simulink model "Model_FOPID_autotuning"  (Simulink 9.2)
settings: Solver=VariableStepAuto  StartTime=0.0  StopTime=100  FixedStep=T_s  MaxStep=1e-3  RelTol=1e-3  EnableMultiTasking=on
values from neighbouring files (symbols this model uses):
  d = step_value    (= 1)    [GUI_ZNFOPID.m]
  disturb_step_time = sim_time*2    (= 200)    [GUI_ZNFOPID.m]
  disturb_step_value = 0.3    [GUI_ZNFOPID.m]
  h = step_value    (= 1)    [GUI_ZNFOPID.m]
  Kp = alpha*Kc    [Function_ZNPID_mu.m]    (also in GUI_ZNFOPID.m = handles.Kp)
  L = 0    [GUI_ZNFOPID.m]
  step_value = 1    [GUI_ZNFOPID.m]
  SW = 0    [GUI_ZNFOPID.m]
  Td = gamma*Tc^mu    [Function_ZNPID_mu.m]    (also in GUI_ZNFOPID.m = handles.Td)
  Ti = beta*Tc    [Function_ZNPID_mu.m]    (also in GUI_ZNFOPID.m = handles.Ti)
libraries: cstblocks x2, powerlib x1
settings Model: Creator=Li Chuang  LastModifiedBy=18764
settings OptimizationCC: InitFltsAndDblsToZero=on
settings DebuggingCC: SaveWithParameterizedLinksMsg=none  SignalResolutionControl=TryResolveAllWithWarning  SolverPrmCheckMsg=warning  MultiTaskDSMMsg=warning  MultiTaskCondExecSysMsg=none  FcnCallInpInsideContextMsg=error  AllowSymbolicDim=off  StateNameClashWarn=none
settings GRTTargetCC: TargetFcnLib=ansi_tfl_tmw.mat  GeneratePreprocessorConditionals=Use local settings

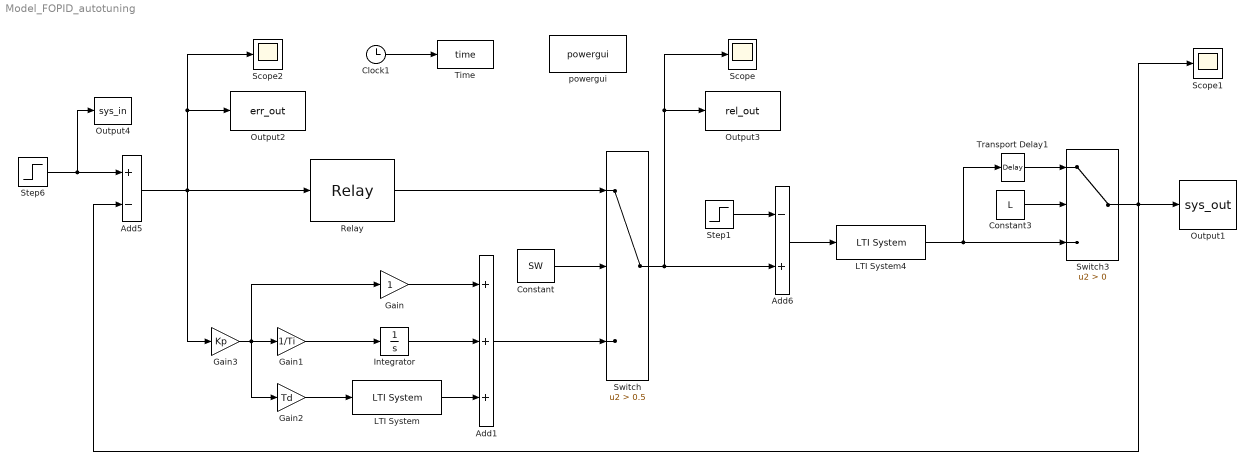
== system Model_FOPID_autotuning ==
  Add1 : Sum  Inputs=+++  SaturateOnIntegerOverflow=on  OutDataTypeStr=Inherit: Same as first input
  Add5 : Sum  Inputs=+-  SaturateOnIntegerOverflow=on  OutDataTypeStr=Inherit: Same as first input
  Add6 : Sum  Inputs=-+  SaturateOnIntegerOverflow=on  OutDataTypeStr=Inherit: Same as first input
  Clock1 : Clock
      settings: Decimation=100
  Constant : Constant  Value=SW
  Constant3 : Constant  Value=L
  Gain : Gain
  Gain1 : Gain  Gain=1/Ti
  Gain2 : Gain  Gain=Td
  Gain3 : Gain  Gain=Kp
  Integrator : Integrator
  LTI System : cstblocks/LTI System  sys=dfo  IC=[]
  LTI System4 : cstblocks/LTI System  sys=Gp  IC=[]
  Output1 : ToWorkspace  VariableName=sys_out  SampleTime=-1
  Output2 : ToWorkspace  VariableName=err_out  SampleTime=-1
  Output3 : ToWorkspace  VariableName=rel_out  SampleTime=-1
  Output4 : ToWorkspace  VariableName=sys_in  SampleTime=-1
  Relay : Relay  OnSwitchValue=d  OffSwitchValue=-d  OnOutputValue=h  OffOutputValue=-h
  Scope : Scope
  Scope1 : Scope
  Scope2 : Scope
  Step1 : Step  Time=disturb_step_time  After=disturb_step_value
  Step6 : Step  Time=0  After=step_value
  Switch : Switch  Criteria=u2 > Threshold  Threshold=0.5
  Switch3 : Switch  Criteria=u2 > Threshold
  Time : ToWorkspace  VariableName=time  SampleTime=-1
  Transport Delay1 : TransportDelay  DelayTime=L
  powergui : powerlib/powergui  Priority=1  SimulationMode=Continuous  SampleTime=50e-6  frequency=60  Iterations=50  frequencyindice=60  Pbase=100e6  ErrMax=1e-4  UnitsV=kV  UnitsW=MW  buscounter=0  FunctionMessages=off  echomessages=off  EnableUseOfTLC=off  CurrentSourceSwitches=off  DisableSnubberDevices=off  DisableRonSwitches=off  DisableVfSwitches=off  DisplayEquations=off  SolverType=Tustin/Backward Euler (TBE)  Interpol=off  ExternalGateDelay=off  methode=off  Ts=100  x0status=blocks  SPID=on  SwTol=0  HookPort=off  RestoreLinks=warning  ResistiveCurrentMeasurement=off  Frange=[0:2:500]  Ylog=off  Xlog=on  ShowGrid=off  save=off  variable=ZData  structure=0  ZoomFFT=off  StartTime=0.0  cycles=1  DisplayStyle=1  fundamental=60  FreqAxis=off  MaxFrequency=1000  frequencyindicesteady=1  RmsSteady=1  display=off
  wires:
  Step6/1 -> Output4/1, Add5/1
  Transport Delay1/1 -> Switch3/1
  LTI System4/1 -> Transport Delay1/1, Switch3/3
  Constant3/1 -> Switch3/2
  Switch3/1 -> Scope1/1, Output1/1, Add5/2
  Relay/1 -> Switch/1
  Add1/1 -> Switch/3
  Switch/1 -> Output3/1, Scope/1, Add6/2
  Step1/1 -> Add6/1
  Add6/1 -> LTI System4/1
  Constant/1 -> Switch/2
  Integrator/1 -> Add1/2
  LTI System/1 -> Add1/3
  Gain/1 -> Add1/1
  Gain1/1 -> Integrator/1
  Gain2/1 -> LTI System/1
  Gain3/1 -> Gain2/1, Gain/1, Gain1/1
  Add5/1 -> Gain3/1, Scope2/1, Output2/1, Relay/1
  Clock1/1 -> Time/1
